simulink model "Final_Tune_of_Bandwidth_PI_Result"  (R2022b)
settings: Solver=FixedStepDiscrete  StartTime=0.0  StopTime=Inf  FixedStep=100e-6  RelTol=1e-3  EnableMultiTasking=on
undefined symbols (not defined in the file): C28x, CPU1, CPU2, CurrentBypassValue, DiscIntNeverNeededParam, Down, GPTRIP1SEL, TZ1, Up
libraries: c2802xlib x20, simulink x16, dspstat3 x10, dspsigops x6, c2837xDlib x5, PID_Lib x5, c280xlib x3, c2000lib x1
(part 2 of 3)

== system Final_Tune_of_Bandwidth_PI_Result/Subsystem1/SVM ==
  Vabc : Inport
  Vdc : Inport  Port=2
  Add : Sum
  Add1 : Sum
  Constant1 : Constant
  Divide : Product  Inputs=*/
  Gain : Gain  Gain=uint32(5000)
  Gain2 : Gain  Gain=0.5
  Gain8 : Gain  Gain=0.5
  Gain9 : Gain  Gain=0.5
  Max : MinMax  Function=max
  Max1 : MinMax
  Saturation : Saturate  UpperLimit=single(2/sqrt(3))  LowerLimit=single(-2/sqrt(3))
  Saturation1 : Saturate  UpperLimit=5000  LowerLimit=0
  Subtract : Sum  Inputs=+-
  Dabc : Outport
  wires:
  Max/1 -> Add/1
  Gain8/1 -> Divide/2
  Add1/1 -> Gain9/1
  Add/1 -> Gain2/1
  Vabc/1 -> Subtract/1, Max1/1, Max/1
  Max1/1 -> Add/2
  Divide/1 -> Saturation/1
  Constant1/1 -> Add1/2
  Gain2/1 -> Subtract/2
  Subtract/1 -> Divide/1
  Gain9/1 -> Gain/1
  Vdc/1 -> Gain8/1
  Saturation/1 -> Add1/1
  Gain/1 -> Saturation1/1
  Saturation1/1 -> Dabc/1

== system Final_Tune_of_Bandwidth_PI_Result/Subsystem1/Start ==
  Data : Inport
  Data_width : Inport  Port=2
  Action Port : ActionPort  ActionPortLabel=if(u1 == 0)
  Bias : Bias  Bias=1  SaturateOnIntegerOverflow=off
  End : Constant  Value=hex2dec('5353')  OutDataTypeStr=uint16
  Mux : Mux  Inputs=2
  Data_out : Outport  VectorParamsAs1DForOutWhenUnconnected=off
  Iteration : Outport  Port=2  VectorParamsAs1DForOutWhenUnconnected=off
  wires:
  End/1 -> Mux/1
  Mux/1 -> Data_out/1
  Data_width/1 -> Bias/1
  Bias/1 -> Iteration/1
  Data/1 -> Mux/2

== system Final_Tune_of_Bandwidth_PI_Result/Subsystem1/Subsystem ==
  PWM1 : Inport
  PWM2 : Inport  Port=2
  PWM3 : Inport  Port=3
  Trip : Inport  Port=4
  Constant12 : Constant  Value=uint32(4999)
  Constant13 : Constant  Value=uint32(0)
  Constant16 : Constant  Value=uint32(4999)
  Constant17 : Constant  Value=uint32(0)
  Constant6 : Constant  Value=uint32(4999)
  Constant7 : Constant  Value=uint32(0)
  Data Type Conversion18 : DataTypeConversion  OutDataTypeStr=uint32  SaturateOnIntegerOverflow=off  RndMeth=Floor
  Data Type Conversion19 : DataTypeConversion  OutDataTypeStr=uint32  SaturateOnIntegerOverflow=off  RndMeth=Floor
  Data Type Conversion5 : DataTypeConversion  OutDataTypeStr=uint32  SaturateOnIntegerOverflow=off  RndMeth=Floor
  From : From
  From1 : From
  From2 : From
  Gain : Gain
  Goto : Goto
  Saturation Dynamic1 : simulink/Discontinuities/Saturation Dynamic  OutMin=[]  OutMax=[]  OutDataTypeStr=Inherit: Same as second input  OutDataType=fixdt(1, 16)  OutScaling=2^-10  DoSatur=off
  Saturation Dynamic2 : simulink/Discontinuities/Saturation Dynamic  OutMin=[]  OutMax=[]  OutDataTypeStr=Inherit: Same as second input  OutDataType=fixdt(1, 16)  OutScaling=2^-10  DoSatur=off
  Saturation Dynamic3 : simulink/Discontinuities/Saturation Dynamic  OutMin=[]  OutMax=[]  OutDataTypeStr=Inherit: Same as second input  OutDataType=fixdt(1, 16)  OutScaling=2^-10  DoSatur=off
  ePWM5 : c2802xlib/ePWM  PwmType=C2000_Type4  useModule=ePWM1  ePWMxLINKTBPRD=Not Linked  periodUnits=Clock cycles  timerSource=Specify via dialog  timerPeriod_clk=5000  timerPeriod_sec=0.0001  tbshadow=Counter equals to zero  countingMode=Up-Down  phaseActiveEnable=Disable  phaseDirection=Count down after sync  phaseActive=0  synchronizationEnable=off  dcaevt1Sync=off  dcbevt1Sync=off  synchronizationOption=Disable  dcbevt1SyncOut=off  dcaevt1SyncOut=off  cmpdSyncOut=off  cmpcSyncOut=off  cmpbSyncOut=off  zeroSyncOut=off  swfSyncOut=off  perSynchronizationOption=Counter equals to period (CTR=PRD)  clockPrescale=1  HSclockPrescale=1  enswap=off  ePWMxAStatus=on  ePWMxAactionLogic1=Do nothing  ePWMxAactionLogic2=Do nothing  ePWMxAactionLogic3=Clear  ePWMxAactionLogic4=Set  ePWMxAactionLogic5=Do nothing  ePWMxAactionLogic6=Do nothing  ePWMxACSFenable=off  ePWMxACSFvalue=Forcing disable  ePWMxASFreload=Zero  ePWMxBStatus=off  ePWMxBactionLogic1=Set  ePWMxBactionLogic2=Clear  ePWMxBactionLogic3=Do nothing  ePWMxBactionLogic4=Do nothing  ePWMxBactionLogic5=Clear  ePWMxBactionLogic6=Set  ePWMxBCSFenable=off  ePWMxBCSFvalue=Forcing disable  ePWMxBSFreload=Zero  ePWNxBOutWay=off  ePWMxLINKCMPA=Not Linked  CMPAUnits=Clock cycles  CMPASource=Input port  CMPAValue_per=50  CMPAValue_clk=0  enCMPAshadow=Counter equals to zero (CTR=Zero)  ePWMxLINKCMPB=Not Linked  CMPBUnits=Clock cycles  CMPBSource=Specify via dialog  CMPBValue_per=50  CMPBValue_clk=0  enCMPBshadow=Counter equals to zero (CTR=Zero)  ePWMxLINKCMPC=Not Linked  CMPCUnits=Clock cycles  CMPCSource=Specify via dialog  CMPCValue_per=50  CMPCValue_clk=0  enCMPCshadow=Counter equals to zero (CTR=Zero)  ePWMxLINKCMPD=Not Linked  CMPDUnits=Clock cycles  CMPDSource=Specify via dialog  CMPDValue_per=50  CMPDValue_clk=32000  enCMPDshadow=Counter equals to zero (CTR=Zero)  enableDBePWMxA=on  enableDBePWMxB=on  enhalfcycle=off  DBpolarity=Active high complementary (AHC)  DBedgeDelay=Positive  DBSource_ePWMxA=ePWMxA  DBSource_ePWMxB=ePWMxA  DBPeriodUnits=Clock cycles  DBperiodSource=Specify via dialog  REDperiod=250  FEDperiod=250  REDperiod_sec=0  FEDperiod_sec=0  LoadModeDBRED=Immediate without using shadow  LoadModeDBFED=Immediate without using shadow  adcstartModuleA=on  adcrequestEventA=First event  adcstartEventA=Digital Compare Module A Event 1 start of conversion (DCAEVT1.soc)  adcstartEventA_type2=Counter equals to period (CTR=PRD)  adcstartModuleB=off  adcrequestEventB=First event  adcstartEventB=Counter equals to zero (CTR=Zero)  adcstartEventB_type2=Counter equals to zero (CTR=Zero)  intEn=off  intPrd=First event  intSel=Counter equals to zero (CTR=Zero)  intSel_type2=Counter equals to zero (CTR=Zero)  hrpe=off  enHRPWM=off  HRPWM_LoadMode=Counter equals to period (CTR=PRD)  HRPWM_CTLMode=Duty or Period control mode  HRPWM_EDGMode=Both edge  hrpeb=off  enHRPWMB=off  HRPWM_LoadModeB=Counter equals to zero (CTR=ZERO)  HRPWM_CTLModeB=Duty or Period control mode  HRPWM_EDGModeB=Both edge  enHRDBRED=off  enHRDBFED=off  enSFO=on  enautoconv=on  chopperEnable=off  chopperFrequency=1  chopperFirstwidth=1  chopperDuty=12.5%  tripZonesource=Input port  tzselOSHT1=off  tzselOSHT2=off  tzselOSHT3=off  tzselOSHDCAEV1=off  tzselOSHDCBEV1=off  tzselCBC1=off  tzselCBC2=off  tzselCBC3=off  tzselCBCDCAEV2=off  tzselCBCDCBEV2=off  tzselOSHT4=off  tzselOSHT5=off  tzselOSHT6=off  tzselCBC4=off  tzselCBC5=off  tzselCBC6=off  enTzOstIntr=off  enTzCbcIntr=off  enTzDCAEVT1Intr=off  enTzDCAEVT2Intr=off  enTzDCBEVT1Intr=off  enTzDCBEVT2Intr=off  ePWMxAforced=Low  ePWMxBforced=Low  DCAEVT1forced=No action  DCBEVT1forced=No action  DCAEVT2forced=No action  DCBEVT2forced=No action  dcah=Trip Zone 1 input (TZ1)  dcal=Trip Zone 2 input (TZ2)  dcbh=Trip Zone 1 input (TZ1)  dcbl=Trip Zone 2 input (TZ2)  dcah_type2=GPTRIP1SEL/(TZ1)  dcal_type2=GPTRIP1SEL/(TZ1)  dcbh_type2=GPTRIP1SEL/(TZ1)  dcbl_type2=GPTRIP1SEL/(TZ1)  gendcaevt1=Event disabled  gendcaevt2=Event disabled  gendcbevt1=Event disabled  gendcbevt2=Event disabled  dcaevt1src=DCAEVT1 with sync  dcaevt2src=DCAEVT2 with sync  dcbevt1src=DCBEVT1 with sync  dcbevt2src=DCBEVT2 with sync  pulsesel=Counter equals to zero (CTR=Zero)  blankinv=off  blankoffset=0  blankwidth=0  evsrcsel=Filtered version of DCAEVT1 (DCAEVT1FILT)  encape=off
  ePWM6 : c2802xlib/ePWM  PwmType=C2000_Type4  useModule=ePWM2  ePWMxLINKTBPRD=Not Linked  periodUnits=Clock cycles  timerSource=Specify via dialog  timerPeriod_clk=5000  timerPeriod_sec=0.0001  tbshadow=Counter equals to zero  countingMode=Up-Down  phaseActiveEnable=Disable  phaseDirection=Count down after sync  phaseActive=0  synchronizationEnable=off  dcaevt1Sync=off  dcbevt1Sync=off  synchronizationOption=Disable  dcbevt1SyncOut=off  dcaevt1SyncOut=off  cmpdSyncOut=off  cmpcSyncOut=off  cmpbSyncOut=off  zeroSyncOut=off  swfSyncOut=off  perSynchronizationOption=Counter equals to period (CTR=PRD)  clockPrescale=1  HSclockPrescale=1  enswap=off  ePWMxAStatus=on  ePWMxAactionLogic1=Do nothing  ePWMxAactionLogic2=Do nothing  ePWMxAactionLogic3=Clear  ePWMxAactionLogic4=Set  ePWMxAactionLogic5=Do nothing  ePWMxAactionLogic6=Do nothing  ePWMxACSFenable=off  ePWMxACSFvalue=Forcing disable  ePWMxASFreload=Zero  ePWMxBStatus=off  ePWMxBactionLogic1=Set  ePWMxBactionLogic2=Clear  ePWMxBactionLogic3=Do nothing  ePWMxBactionLogic4=Do nothing  ePWMxBactionLogic5=Clear  ePWMxBactionLogic6=Set  ePWMxBCSFenable=off  ePWMxBCSFvalue=Forcing disable  ePWMxBSFreload=Zero  ePWNxBOutWay=off  ePWMxLINKCMPA=Not Linked  CMPAUnits=Clock cycles  CMPASource=Input port  CMPAValue_per=50  CMPAValue_clk=0  enCMPAshadow=Counter equals to zero (CTR=Zero)  ePWMxLINKCMPB=Not Linked  CMPBUnits=Clock cycles  CMPBSource=Specify via dialog  CMPBValue_per=50  CMPBValue_clk=0  enCMPBshadow=Counter equals to zero (CTR=Zero)  ePWMxLINKCMPC=Not Linked  CMPCUnits=Clock cycles  CMPCSource=Specify via dialog  CMPCValue_per=50  CMPCValue_clk=0  enCMPCshadow=Counter equals to zero (CTR=Zero)  ePWMxLINKCMPD=Not Linked  CMPDUnits=Clock cycles  CMPDSource=Specify via dialog  CMPDValue_per=50  CMPDValue_clk=32000  enCMPDshadow=Counter equals to zero (CTR=Zero)  enableDBePWMxA=on  enableDBePWMxB=on  enhalfcycle=off  DBpolarity=Active high complementary (AHC)  DBedgeDelay=Positive  DBSource_ePWMxA=ePWMxA  DBSource_ePWMxB=ePWMxA  DBPeriodUnits=Clock cycles  DBperiodSource=Specify via dialog  REDperiod=250  FEDperiod=250  REDperiod_sec=0  FEDperiod_sec=0  LoadModeDBRED=Immediate without using shadow  LoadModeDBFED=Immediate without using shadow  adcstartModuleA=off  adcrequestEventA=First event  adcstartEventA=Digital Compare Module A Event 1 start of conversion (DCAEVT1.soc)  adcstartEventA_type2=Counter equals to zero (CTR=Zero)  adcstartModuleB=off  adcrequestEventB=First event  adcstartEventB=Counter equals to zero (CTR=Zero)  adcstartEventB_type2=Counter equals to zero (CTR=Zero)  intEn=off  intPrd=First event  intSel=Counter equals to zero (CTR=Zero)  intSel_type2=Counter equals to zero (CTR=Zero)  hrpe=off  enHRPWM=off  HRPWM_LoadMode=Counter equals to period (CTR=PRD)  HRPWM_CTLMode=Duty or Period control mode  HRPWM_EDGMode=Both edge  hrpeb=off  enHRPWMB=off  HRPWM_LoadModeB=Counter equals to zero (CTR=ZERO)  HRPWM_CTLModeB=Duty or Period control mode  HRPWM_EDGModeB=Both edge  enHRDBRED=off  enHRDBFED=off  enSFO=on  enautoconv=on  chopperEnable=off  chopperFrequency=1  chopperFirstwidth=1  chopperDuty=12.5%  tripZonesource=Input port  tzselOSHT1=off  tzselOSHT2=off  tzselOSHT3=off  tzselOSHDCAEV1=off  tzselOSHDCBEV1=off  tzselCBC1=off  tzselCBC2=off  tzselCBC3=off  tzselCBCDCAEV2=off  tzselCBCDCBEV2=off  tzselOSHT4=off  tzselOSHT5=off  tzselOSHT6=off  tzselCBC4=off  tzselCBC5=off  tzselCBC6=off  enTzOstIntr=off  enTzCbcIntr=off  enTzDCAEVT1Intr=off  enTzDCAEVT2Intr=off  enTzDCBEVT1Intr=off  enTzDCBEVT2Intr=off  ePWMxAforced=Low  ePWMxBforced=Low  DCAEVT1forced=No action  DCBEVT1forced=No action  DCAEVT2forced=No action  DCBEVT2forced=No action  dcah=Trip Zone 1 input (TZ1)  dcal=Trip Zone 2 input (TZ2)  dcbh=Trip Zone 1 input (TZ1)  dcbl=Trip Zone 2 input (TZ2)  dcah_type2=GPTRIP1SEL/(TZ1)  dcal_type2=GPTRIP1SEL/(TZ1)  dcbh_type2=GPTRIP1SEL/(TZ1)  dcbl_type2=GPTRIP1SEL/(TZ1)  gendcaevt1=Event disabled  gendcaevt2=Event disabled  gendcbevt1=Event disabled  gendcbevt2=Event disabled  dcaevt1src=DCAEVT1 with sync  dcaevt2src=DCAEVT2 with sync  dcbevt1src=DCBEVT1 with sync  dcbevt2src=DCBEVT2 with sync  pulsesel=Counter equals to zero (CTR=Zero)  blankinv=off  blankoffset=0  blankwidth=0  evsrcsel=Filtered version of DCAEVT1 (DCAEVT1FILT)  encape=off
  ePWM7 : c2802xlib/ePWM  PwmType=C2000_Type4  useModule=ePWM3  ePWMxLINKTBPRD=Not Linked  periodUnits=Clock cycles  timerSource=Specify via dialog  timerPeriod_clk=5000  timerPeriod_sec=0.0001  tbshadow=Counter equals to zero  countingMode=Up-Down  phaseActiveEnable=Disable  phaseDirection=Count down after sync  phaseActive=0  synchronizationEnable=off  dcaevt1Sync=off  dcbevt1Sync=off  synchronizationOption=Disable  dcbevt1SyncOut=off  dcaevt1SyncOut=off  cmpdSyncOut=off  cmpcSyncOut=off  cmpbSyncOut=off  zeroSyncOut=off  swfSyncOut=off  perSynchronizationOption=Counter equals to period (CTR=PRD)  clockPrescale=1  HSclockPrescale=1  enswap=off  ePWMxAStatus=on  ePWMxAactionLogic1=Do nothing  ePWMxAactionLogic2=Do nothing  ePWMxAactionLogic3=Clear  ePWMxAactionLogic4=Set  ePWMxAactionLogic5=Do nothing  ePWMxAactionLogic6=Do nothing  ePWMxACSFenable=off  ePWMxACSFvalue=Forcing disable  ePWMxASFreload=Zero  ePWMxBStatus=off  ePWMxBactionLogic1=Set  ePWMxBactionLogic2=Clear  ePWMxBactionLogic3=Do nothing  ePWMxBactionLogic4=Do nothing  ePWMxBactionLogic5=Clear  ePWMxBactionLogic6=Set  ePWMxBCSFenable=off  ePWMxBCSFvalue=Forcing disable  ePWMxBSFreload=Zero  ePWNxBOutWay=off  ePWMxLINKCMPA=Not Linked  CMPAUnits=Clock cycles  CMPASource=Input port  CMPAValue_per=50  CMPAValue_clk=0  enCMPAshadow=Counter equals to zero (CTR=Zero)  ePWMxLINKCMPB=Not Linked  CMPBUnits=Clock cycles  CMPBSource=Specify via dialog  CMPBValue_per=50  CMPBValue_clk=0  enCMPBshadow=Counter equals to zero (CTR=Zero)  ePWMxLINKCMPC=Not Linked  CMPCUnits=Clock cycles  CMPCSource=Specify via dialog  CMPCValue_per=50  CMPCValue_clk=0  enCMPCshadow=Counter equals to zero (CTR=Zero)  ePWMxLINKCMPD=Not Linked  CMPDUnits=Clock cycles  CMPDSource=Specify via dialog  CMPDValue_per=50  CMPDValue_clk=32000  enCMPDshadow=Counter equals to zero (CTR=Zero)  enableDBePWMxA=on  enableDBePWMxB=on  enhalfcycle=off  DBpolarity=Active high complementary (AHC)  DBedgeDelay=Positive  DBSource_ePWMxA=ePWMxA  DBSource_ePWMxB=ePWMxA  DBPeriodUnits=Clock cycles  DBperiodSource=Specify via dialog  REDperiod=250  FEDperiod=250  REDperiod_sec=0  FEDperiod_sec=0  LoadModeDBRED=Immediate without using shadow  LoadModeDBFED=Immediate without using shadow  adcstartModuleA=off  adcrequestEventA=First event  adcstartEventA=Digital Compare Module A Event 1 start of conversion (DCAEVT1.soc)  adcstartEventA_type2=Counter equals to zero (CTR=Zero)  adcstartModuleB=off  adcrequestEventB=First event  adcstartEventB=Counter equals to zero (CTR=Zero)  adcstartEventB_type2=Counter equals to zero (CTR=Zero)  intEn=off  intPrd=First event  intSel=Counter equals to zero (CTR=Zero)  intSel_type2=Counter equals to zero (CTR=Zero)  hrpe=off  enHRPWM=off  HRPWM_LoadMode=Counter equals to period (CTR=PRD)  HRPWM_CTLMode=Duty or Period control mode  HRPWM_EDGMode=Both edge  hrpeb=off  enHRPWMB=off  HRPWM_LoadModeB=Counter equals to zero (CTR=ZERO)  HRPWM_CTLModeB=Duty or Period control mode  HRPWM_EDGModeB=Both edge  enHRDBRED=off  enHRDBFED=off  enSFO=on  enautoconv=on  chopperEnable=off  chopperFrequency=1  chopperFirstwidth=1  chopperDuty=12.5%  tripZonesource=Input port  tzselOSHT1=off  tzselOSHT2=off  tzselOSHT3=off  tzselOSHDCAEV1=off  tzselOSHDCBEV1=off  tzselCBC1=off  tzselCBC2=off  tzselCBC3=off  tzselCBCDCAEV2=off  tzselCBCDCBEV2=off  tzselOSHT4=off  tzselOSHT5=off  tzselOSHT6=off  tzselCBC4=off  tzselCBC5=off  tzselCBC6=off  enTzOstIntr=off  enTzCbcIntr=off  enTzDCAEVT1Intr=off  enTzDCAEVT2Intr=off  enTzDCBEVT1Intr=off  enTzDCBEVT2Intr=off  ePWMxAforced=Low  ePWMxBforced=Low  DCAEVT1forced=No action  DCBEVT1forced=No action  DCAEVT2forced=No action  DCBEVT2forced=No action  dcah=Trip Zone 1 input (TZ1)  dcal=Trip Zone 2 input (TZ2)  dcbh=Trip Zone 1 input (TZ1)  dcbl=Trip Zone 2 input (TZ2)  dcah_type2=GPTRIP1SEL/(TZ1)  dcal_type2=GPTRIP1SEL/(TZ1)  dcbh_type2=GPTRIP1SEL/(TZ1)  dcbl_type2=GPTRIP1SEL/(TZ1)  gendcaevt1=Event disabled  gendcaevt2=Event disabled  gendcbevt1=Event disabled  gendcbevt2=Event disabled  dcaevt1src=DCAEVT1 with sync  dcaevt2src=DCAEVT2 with sync  dcbevt1src=DCBEVT1 with sync  dcbevt2src=DCBEVT2 with sync  pulsesel=Counter equals to zero (CTR=Zero)  blankinv=off  blankoffset=0  blankwidth=0  evsrcsel=Filtered version of DCAEVT1 (DCAEVT1FILT)  encape=off
  wires:
  Data Type Conversion5/1 -> ePWM5/1
  Constant13/1 -> Saturation Dynamic3/3
  Constant6/1 -> Saturation Dynamic1/1
  Constant12/1 -> Saturation Dynamic3/1
  Constant7/1 -> Saturation Dynamic1/3
  Saturation Dynamic1/1 -> Data Type Conversion5/1
  Constant16/1 -> Saturation Dynamic2/1
  Data Type Conversion18/1 -> ePWM6/1
  Data Type Conversion19/1 -> ePWM7/1
  Saturation Dynamic3/1 -> Data Type Conversion19/1
  Constant17/1 -> Saturation Dynamic2/3
  Saturation Dynamic2/1 -> Data Type Conversion18/1
  PWM1/1 -> Saturation Dynamic1/2
  PWM3/1 -> Saturation Dynamic3/2
  PWM2/1 -> Saturation Dynamic2/2
  From/1 -> ePWM5/2
  From1/1 -> ePWM6/2
  From2/1 -> ePWM7/2
  Trip/1 -> Gain/1
  Gain/1 -> Goto/1

== system Final_Tune_of_Bandwidth_PI_Result/Subsystem1/Subsystem1 ==
  In1 : Inport
  In2 : Inport  Port=2
  Enable : EnablePort  StatesWhenEnabling=reset
  Add : Sum
  Add3 : Sum
  Bus Creator : BusCreator  Inputs=2
  Bus Selector1 : BusSelector  OutputSignals=signal1,signal2
  CodeGeneration : Subsystem  TreatAsAtomicUnit=on
  Constant3 : Constant  Value=10  OutDataTypeStr=single
  Counter Limited : simulink/Sources/Counter Limited  uplimit=599  tsamp=-1
  Data : Subsystem  TreatAsAtomicUnit=on
  Data_Conditioning : Subsystem
  End : Subsystem  TreatAsAtomicUnit=on
  Gain6 : Gain  Gain=1000  OutDataTypeStr=single
  Gain7 : Gain  Gain=1000  OutDataTypeStr=single
  If : If  IfExpression=u1 == 0  ElseIfExpressions=u1 == 599
  Merge : Merge  Inputs=3
  Merge1 : Merge  Inputs=3
  Mux : Mux  Inputs=2
  Mux1 : Mux  Inputs=2
  Start : Subsystem  TreatAsAtomicUnit=on
  Width : Width  OutDataTypeMode=All ports same datatype  DataType=uint16
  wires:
  Start/2(Iteration) -> Merge1/1
  Constant3/1 -> Add/2, Add3/1
  Counter Limited/1 -> If/1
  Data_Conditioning/1(Out1) -> Width/1, Start/1(Data), End/1(Data), Data/1(Data)
  End/1(Data_out) -> Merge/2
  End/2(Iteration) -> Merge1/2
  If/3 -> Data/Action
  Add/1 -> Gain6/1
  Data/2(Iteration) -> Merge1/3
  Merge1/1 -> Mux/2  "SCI_Tx_Iteration"
  Bus Selector1/1 -> Add/1  "<signal1>"
  Start/1(Data_out) -> Merge/1
  Add3/1 -> Gain7/1
  Mux1/1 -> Data_Conditioning/1(In1)
  In1/1 -> Bus Creator/1
  Merge/1 -> Mux/1  "SCI_Tx_Data"
  If/2 -> End/Action
  Data/1(Data_out) -> Merge/3
  Bus Creator/1 -> Bus Selector1/1
  Width/1 -> Start/2(Data_width), Data/2(Data_width), End/2(Data_width)
  Mux/1 -> CodeGeneration/1(Input)
  In2/1 -> Bus Creator/2
  Gain7/1 -> Mux1/2
  Bus Selector1/2 -> Add3/2  "<signal2>"
  If/1 -> Start/Action
  Gain6/1 -> Mux1/1

== system Final_Tune_of_Bandwidth_PI_Result/Subsystem1/Subsystem2 ==
  PWM1 : Inport
  PWM2 : Inport  Port=2
  PWM3 : Inport  Port=3
  Trip : Inport  Port=4
  Constant12 : Constant  Value=uint32(4999)
  Constant13 : Constant  Value=uint32(0)
  Constant16 : Constant  Value=uint32(4999)
  Constant17 : Constant  Value=uint32(0)
  Constant6 : Constant  Value=uint32(4999)
  Constant7 : Constant  Value=uint32(0)
  Data Type Conversion18 : DataTypeConversion  OutDataTypeStr=uint32  SaturateOnIntegerOverflow=off  RndMeth=Floor
  Data Type Conversion19 : DataTypeConversion  OutDataTypeStr=uint32  SaturateOnIntegerOverflow=off  RndMeth=Floor
  Data Type Conversion5 : DataTypeConversion  OutDataTypeStr=uint32  SaturateOnIntegerOverflow=off  RndMeth=Floor
  From : From
  From1 : From
  From2 : From
  Gain : Gain
  Goto : Goto
  Saturation Dynamic1 : simulink/Discontinuities/Saturation Dynamic  OutMin=[]  OutMax=[]  OutDataTypeStr=Inherit: Same as second input  OutDataType=fixdt(1, 16)  OutScaling=2^-10  DoSatur=off
  Saturation Dynamic2 : simulink/Discontinuities/Saturation Dynamic  OutMin=[]  OutMax=[]  OutDataTypeStr=Inherit: Same as second input  OutDataType=fixdt(1, 16)  OutScaling=2^-10  DoSatur=off
  Saturation Dynamic3 : simulink/Discontinuities/Saturation Dynamic  OutMin=[]  OutMax=[]  OutDataTypeStr=Inherit: Same as second input  OutDataType=fixdt(1, 16)  OutScaling=2^-10  DoSatur=off
  ePWM5 : c2802xlib/ePWM  PwmType=C2000_Type4  useModule=ePWM1  ePWMxLINKTBPRD=Not Linked  periodUnits=Clock cycles  timerSource=Specify via dialog  timerPeriod_clk=5000  timerPeriod_sec=0.0001  tbshadow=Counter equals to zero  countingMode=Up-Down  phaseActiveEnable=Disable  phaseDirection=Count down after sync  phaseActive=0  synchronizationEnable=off  dcaevt1Sync=off  dcbevt1Sync=off  synchronizationOption=Disable  dcbevt1SyncOut=off  dcaevt1SyncOut=off  cmpdSyncOut=off  cmpcSyncOut=off  cmpbSyncOut=off  zeroSyncOut=off  swfSyncOut=off  perSynchronizationOption=Counter equals to period (CTR=PRD)  clockPrescale=1  HSclockPrescale=1  enswap=off  ePWMxAStatus=on  ePWMxAactionLogic1=Do nothing  ePWMxAactionLogic2=Do nothing  ePWMxAactionLogic3=Clear  ePWMxAactionLogic4=Set  ePWMxAactionLogic5=Do nothing  ePWMxAactionLogic6=Do nothing  ePWMxACSFenable=off  ePWMxACSFvalue=Forcing disable  ePWMxASFreload=Zero  ePWMxBStatus=off  ePWMxBactionLogic1=Set  ePWMxBactionLogic2=Clear  ePWMxBactionLogic3=Do nothing  ePWMxBactionLogic4=Do nothing  ePWMxBactionLogic5=Clear  ePWMxBactionLogic6=Set  ePWMxBCSFenable=off  ePWMxBCSFvalue=Forcing disable  ePWMxBSFreload=Zero  ePWNxBOutWay=off  ePWMxLINKCMPA=Not Linked  CMPAUnits=Clock cycles  CMPASource=Input port  CMPAValue_per=50  CMPAValue_clk=0  enCMPAshadow=Counter equals to zero (CTR=Zero)  ePWMxLINKCMPB=Not Linked  CMPBUnits=Clock cycles  CMPBSource=Specify via dialog  CMPBValue_per=50  CMPBValue_clk=0  enCMPBshadow=Counter equals to zero (CTR=Zero)  ePWMxLINKCMPC=Not Linked  CMPCUnits=Clock cycles  CMPCSource=Specify via dialog  CMPCValue_per=50  CMPCValue_clk=0  enCMPCshadow=Counter equals to zero (CTR=Zero)  ePWMxLINKCMPD=Not Linked  CMPDUnits=Clock cycles  CMPDSource=Specify via dialog  CMPDValue_per=50  CMPDValue_clk=32000  enCMPDshadow=Counter equals to zero (CTR=Zero)  enableDBePWMxA=on  enableDBePWMxB=on  enhalfcycle=off  DBpolarity=Active high complementary (AHC)  DBedgeDelay=Positive  DBSource_ePWMxA=ePWMxA  DBSource_ePWMxB=ePWMxA  DBPeriodUnits=Seconds  DBperiodSource=Specify via dialog  REDperiod=250  FEDperiod=250  REDperiod_sec=500e-9  FEDperiod_sec=500e-9  LoadModeDBRED=Immediate without using shadow  LoadModeDBFED=Immediate without using shadow  adcstartModuleA=on  adcrequestEventA=First event  adcstartEventA=Digital Compare Module A Event 1 start of conversion (DCAEVT1.soc)  adcstartEventA_type2=Counter equals to period (CTR=PRD)  adcstartModuleB=off  adcrequestEventB=First event  adcstartEventB=Counter equals to zero (CTR=Zero)  adcstartEventB_type2=Counter equals to zero (CTR=Zero)  intEn=off  intPrd=First event  intSel=Counter equals to zero (CTR=Zero)  intSel_type2=Counter equals to zero (CTR=Zero)  hrpe=off  enHRPWM=off  HRPWM_LoadMode=Counter equals to period (CTR=PRD)  HRPWM_CTLMode=Duty or Period control mode  HRPWM_EDGMode=Both edge  hrpeb=off  enHRPWMB=off  HRPWM_LoadModeB=Counter equals to zero (CTR=ZERO)  HRPWM_CTLModeB=Duty or Period control mode  HRPWM_EDGModeB=Both edge  enHRDBRED=off  enHRDBFED=off  enSFO=on  enautoconv=on  chopperEnable=off  chopperFrequency=1  chopperFirstwidth=1  chopperDuty=12.5%  tripZonesource=Input port  tzselOSHT1=off  tzselOSHT2=off  tzselOSHT3=off  tzselOSHDCAEV1=off  tzselOSHDCBEV1=off  tzselCBC1=off  tzselCBC2=off  tzselCBC3=off  tzselCBCDCAEV2=off  tzselCBCDCBEV2=off  tzselOSHT4=off  tzselOSHT5=off  tzselOSHT6=off  tzselCBC4=off  tzselCBC5=off  tzselCBC6=off  enTzOstIntr=off  enTzCbcIntr=off  enTzDCAEVT1Intr=off  enTzDCAEVT2Intr=off  enTzDCBEVT1Intr=off  enTzDCBEVT2Intr=off  ePWMxAforced=Low  ePWMxBforced=Low  DCAEVT1forced=No action  DCBEVT1forced=No action  DCAEVT2forced=No action  DCBEVT2forced=No action  dcah=Trip Zone 1 input (TZ1)  dcal=Trip Zone 2 input (TZ2)  dcbh=Trip Zone 1 input (TZ1)  dcbl=Trip Zone 2 input (TZ2)  dcah_type2=GPTRIP1SEL/(TZ1)  dcal_type2=GPTRIP1SEL/(TZ1)  dcbh_type2=GPTRIP1SEL/(TZ1)  dcbl_type2=GPTRIP1SEL/(TZ1)  gendcaevt1=Event disabled  gendcaevt2=Event disabled  gendcbevt1=Event disabled  gendcbevt2=Event disabled  dcaevt1src=DCAEVT1 with sync  dcaevt2src=DCAEVT2 with sync  dcbevt1src=DCBEVT1 with sync  dcbevt2src=DCBEVT2 with sync  pulsesel=Counter equals to zero (CTR=Zero)  blankinv=off  blankoffset=0  blankwidth=0  evsrcsel=Filtered version of DCAEVT1 (DCAEVT1FILT)  encape=off
  ePWM6 : c2802xlib/ePWM  PwmType=C2000_Type4  useModule=ePWM2  ePWMxLINKTBPRD=Not Linked  periodUnits=Clock cycles  timerSource=Specify via dialog  timerPeriod_clk=5000  timerPeriod_sec=0.0001  tbshadow=Counter equals to zero  countingMode=Up-Down  phaseActiveEnable=Disable  phaseDirection=Count down after sync  phaseActive=0  synchronizationEnable=off  dcaevt1Sync=off  dcbevt1Sync=off  synchronizationOption=Disable  dcbevt1SyncOut=off  dcaevt1SyncOut=off  cmpdSyncOut=off  cmpcSyncOut=off  cmpbSyncOut=off  zeroSyncOut=off  swfSyncOut=off  perSynchronizationOption=Counter equals to period (CTR=PRD)  clockPrescale=1  HSclockPrescale=1  enswap=off  ePWMxAStatus=on  ePWMxAactionLogic1=Do nothing  ePWMxAactionLogic2=Do nothing  ePWMxAactionLogic3=Clear  ePWMxAactionLogic4=Set  ePWMxAactionLogic5=Do nothing  ePWMxAactionLogic6=Do nothing  ePWMxACSFenable=off  ePWMxACSFvalue=Forcing disable  ePWMxASFreload=Zero  ePWMxBStatus=off  ePWMxBactionLogic1=Set  ePWMxBactionLogic2=Clear  ePWMxBactionLogic3=Do nothing  ePWMxBactionLogic4=Do nothing  ePWMxBactionLogic5=Clear  ePWMxBactionLogic6=Set  ePWMxBCSFenable=off  ePWMxBCSFvalue=Forcing disable  ePWMxBSFreload=Zero  ePWNxBOutWay=off  ePWMxLINKCMPA=Not Linked  CMPAUnits=Clock cycles  CMPASource=Input port  CMPAValue_per=50  CMPAValue_clk=0  enCMPAshadow=Counter equals to zero (CTR=Zero)  ePWMxLINKCMPB=Not Linked  CMPBUnits=Clock cycles  CMPBSource=Specify via dialog  CMPBValue_per=50  CMPBValue_clk=0  enCMPBshadow=Counter equals to zero (CTR=Zero)  ePWMxLINKCMPC=Not Linked  CMPCUnits=Clock cycles  CMPCSource=Specify via dialog  CMPCValue_per=50  CMPCValue_clk=0  enCMPCshadow=Counter equals to zero (CTR=Zero)  ePWMxLINKCMPD=Not Linked  CMPDUnits=Clock cycles  CMPDSource=Specify via dialog  CMPDValue_per=50  CMPDValue_clk=32000  enCMPDshadow=Counter equals to zero (CTR=Zero)  enableDBePWMxA=on  enableDBePWMxB=on  enhalfcycle=off  DBpolarity=Active high complementary (AHC)  DBedgeDelay=Positive  DBSource_ePWMxA=ePWMxA  DBSource_ePWMxB=ePWMxA  DBPeriodUnits=Seconds  DBperiodSource=Specify via dialog  REDperiod=250  FEDperiod=250  REDperiod_sec=500e-9  FEDperiod_sec=500e-9  LoadModeDBRED=Immediate without using shadow  LoadModeDBFED=Immediate without using shadow  adcstartModuleA=off  adcrequestEventA=First event  adcstartEventA=Digital Compare Module A Event 1 start of conversion (DCAEVT1.soc)  adcstartEventA_type2=Counter equals to zero (CTR=Zero)  adcstartModuleB=off  adcrequestEventB=First event  adcstartEventB=Counter equals to zero (CTR=Zero)  adcstartEventB_type2=Counter equals to zero (CTR=Zero)  intEn=off  intPrd=First event  intSel=Counter equals to zero (CTR=Zero)  intSel_type2=Counter equals to zero (CTR=Zero)  hrpe=off  enHRPWM=off  HRPWM_LoadMode=Counter equals to period (CTR=PRD)  HRPWM_CTLMode=Duty or Period control mode  HRPWM_EDGMode=Both edge  hrpeb=off  enHRPWMB=off  HRPWM_LoadModeB=Counter equals to zero (CTR=ZERO)  HRPWM_CTLModeB=Duty or Period control mode  HRPWM_EDGModeB=Both edge  enHRDBRED=off  enHRDBFED=off  enSFO=on  enautoconv=on  chopperEnable=off  chopperFrequency=1  chopperFirstwidth=1  chopperDuty=12.5%  tripZonesource=Input port  tzselOSHT1=off  tzselOSHT2=off  tzselOSHT3=off  tzselOSHDCAEV1=off  tzselOSHDCBEV1=off  tzselCBC1=off  tzselCBC2=off  tzselCBC3=off  tzselCBCDCAEV2=off  tzselCBCDCBEV2=off  tzselOSHT4=off  tzselOSHT5=off  tzselOSHT6=off  tzselCBC4=off  tzselCBC5=off  tzselCBC6=off  enTzOstIntr=off  enTzCbcIntr=off  enTzDCAEVT1Intr=off  enTzDCAEVT2Intr=off  enTzDCBEVT1Intr=off  enTzDCBEVT2Intr=off  ePWMxAforced=Low  ePWMxBforced=Low  DCAEVT1forced=No action  DCBEVT1forced=No action  DCAEVT2forced=No action  DCBEVT2forced=No action  dcah=Trip Zone 1 input (TZ1)  dcal=Trip Zone 2 input (TZ2)  dcbh=Trip Zone 1 input (TZ1)  dcbl=Trip Zone 2 input (TZ2)  dcah_type2=GPTRIP1SEL/(TZ1)  dcal_type2=GPTRIP1SEL/(TZ1)  dcbh_type2=GPTRIP1SEL/(TZ1)  dcbl_type2=GPTRIP1SEL/(TZ1)  gendcaevt1=Event disabled  gendcaevt2=Event disabled  gendcbevt1=Event disabled  gendcbevt2=Event disabled  dcaevt1src=DCAEVT1 with sync  dcaevt2src=DCAEVT2 with sync  dcbevt1src=DCBEVT1 with sync  dcbevt2src=DCBEVT2 with sync  pulsesel=Counter equals to zero (CTR=Zero)  blankinv=off  blankoffset=0  blankwidth=0  evsrcsel=Filtered version of DCAEVT1 (DCAEVT1FILT)  encape=off
  ePWM7 : c2802xlib/ePWM  PwmType=C2000_Type4  useModule=ePWM3  ePWMxLINKTBPRD=Not Linked  periodUnits=Clock cycles  timerSource=Specify via dialog  timerPeriod_clk=5000  timerPeriod_sec=0.0001  tbshadow=Counter equals to zero  countingMode=Up-Down  phaseActiveEnable=Disable  phaseDirection=Count down after sync  phaseActive=0  synchronizationEnable=off  dcaevt1Sync=off  dcbevt1Sync=off  synchronizationOption=Disable  dcbevt1SyncOut=off  dcaevt1SyncOut=off  cmpdSyncOut=off  cmpcSyncOut=off  cmpbSyncOut=off  zeroSyncOut=off  swfSyncOut=off  perSynchronizationOption=Counter equals to period (CTR=PRD)  clockPrescale=1  HSclockPrescale=1  enswap=off  ePWMxAStatus=on  ePWMxAactionLogic1=Do nothing  ePWMxAactionLogic2=Do nothing  ePWMxAactionLogic3=Clear  ePWMxAactionLogic4=Set  ePWMxAactionLogic5=Do nothing  ePWMxAactionLogic6=Do nothing  ePWMxACSFenable=off  ePWMxACSFvalue=Forcing disable  ePWMxASFreload=Zero  ePWMxBStatus=off  ePWMxBactionLogic1=Set  ePWMxBactionLogic2=Clear  ePWMxBactionLogic3=Do nothing  ePWMxBactionLogic4=Do nothing  ePWMxBactionLogic5=Clear  ePWMxBactionLogic6=Set  ePWMxBCSFenable=off  ePWMxBCSFvalue=Forcing disable  ePWMxBSFreload=Zero  ePWNxBOutWay=off  ePWMxLINKCMPA=Not Linked  CMPAUnits=Clock cycles  CMPASource=Input port  CMPAValue_per=50  CMPAValue_clk=0  enCMPAshadow=Counter equals to zero (CTR=Zero)  ePWMxLINKCMPB=Not Linked  CMPBUnits=Clock cycles  CMPBSource=Specify via dialog  CMPBValue_per=50  CMPBValue_clk=0  enCMPBshadow=Counter equals to zero (CTR=Zero)  ePWMxLINKCMPC=Not Linked  CMPCUnits=Clock cycles  CMPCSource=Specify via dialog  CMPCValue_per=50  CMPCValue_clk=0  enCMPCshadow=Counter equals to zero (CTR=Zero)  ePWMxLINKCMPD=Not Linked  CMPDUnits=Clock cycles  CMPDSource=Specify via dialog  CMPDValue_per=50  CMPDValue_clk=32000  enCMPDshadow=Counter equals to zero (CTR=Zero)  enableDBePWMxA=on  enableDBePWMxB=on  enhalfcycle=off  DBpolarity=Active high complementary (AHC)  DBedgeDelay=Positive  DBSource_ePWMxA=ePWMxA  DBSource_ePWMxB=ePWMxA  DBPeriodUnits=Seconds  DBperiodSource=Specify via dialog  REDperiod=250  FEDperiod=250  REDperiod_sec=500e-9  FEDperiod_sec=500e-9  LoadModeDBRED=Immediate without using shadow  LoadModeDBFED=Immediate without using shadow  adcstartModuleA=off  adcrequestEventA=First event  adcstartEventA=Digital Compare Module A Event 1 start of conversion (DCAEVT1.soc)  adcstartEventA_type2=Counter equals to zero (CTR=Zero)  adcstartModuleB=off  adcrequestEventB=First event  adcstartEventB=Counter equals to zero (CTR=Zero)  adcstartEventB_type2=Counter equals to zero (CTR=Zero)  intEn=off  intPrd=First event  intSel=Counter equals to zero (CTR=Zero)  intSel_type2=Counter equals to zero (CTR=Zero)  hrpe=off  enHRPWM=off  HRPWM_LoadMode=Counter equals to period (CTR=PRD)  HRPWM_CTLMode=Duty or Period control mode  HRPWM_EDGMode=Both edge  hrpeb=off  enHRPWMB=off  HRPWM_LoadModeB=Counter equals to zero (CTR=ZERO)  HRPWM_CTLModeB=Duty or Period control mode  HRPWM_EDGModeB=Both edge  enHRDBRED=off  enHRDBFED=off  enSFO=on  enautoconv=on  chopperEnable=off  chopperFrequency=1  chopperFirstwidth=1  chopperDuty=12.5%  tripZonesource=Input port  tzselOSHT1=off  tzselOSHT2=off  tzselOSHT3=off  tzselOSHDCAEV1=off  tzselOSHDCBEV1=off  tzselCBC1=off  tzselCBC2=off  tzselCBC3=off  tzselCBCDCAEV2=off  tzselCBCDCBEV2=off  tzselOSHT4=off  tzselOSHT5=off  tzselOSHT6=off  tzselCBC4=off  tzselCBC5=off  tzselCBC6=off  enTzOstIntr=off  enTzCbcIntr=off  enTzDCAEVT1Intr=off  enTzDCAEVT2Intr=off  enTzDCBEVT1Intr=off  enTzDCBEVT2Intr=off  ePWMxAforced=Low  ePWMxBforced=Low  DCAEVT1forced=No action  DCBEVT1forced=No action  DCAEVT2forced=No action  DCBEVT2forced=No action  dcah=Trip Zone 1 input (TZ1)  dcal=Trip Zone 2 input (TZ2)  dcbh=Trip Zone 1 input (TZ1)  dcbl=Trip Zone 2 input (TZ2)  dcah_type2=GPTRIP1SEL/(TZ1)  dcal_type2=GPTRIP1SEL/(TZ1)  dcbh_type2=GPTRIP1SEL/(TZ1)  dcbl_type2=GPTRIP1SEL/(TZ1)  gendcaevt1=Event disabled  gendcaevt2=Event disabled  gendcbevt1=Event disabled  gendcbevt2=Event disabled  dcaevt1src=DCAEVT1 with sync  dcaevt2src=DCAEVT2 with sync  dcbevt1src=DCBEVT1 with sync  dcbevt2src=DCBEVT2 with sync  pulsesel=Counter equals to zero (CTR=Zero)  blankinv=off  blankoffset=0  blankwidth=0  evsrcsel=Filtered version of DCAEVT1 (DCAEVT1FILT)  encape=off
  wires:
  Data Type Conversion5/1 -> ePWM5/1
  Constant13/1 -> Saturation Dynamic3/3
  Constant6/1 -> Saturation Dynamic1/1
  Constant12/1 -> Saturation Dynamic3/1
  Constant7/1 -> Saturation Dynamic1/3
  Saturation Dynamic1/1 -> Data Type Conversion5/1
  Constant16/1 -> Saturation Dynamic2/1
  Data Type Conversion18/1 -> ePWM6/1
  Data Type Conversion19/1 -> ePWM7/1
  Saturation Dynamic3/1 -> Data Type Conversion19/1
  Constant17/1 -> Saturation Dynamic2/3
  Saturation Dynamic2/1 -> Data Type Conversion18/1
  PWM1/1 -> Saturation Dynamic1/2
  PWM3/1 -> Saturation Dynamic3/2
  PWM2/1 -> Saturation Dynamic2/2
  From/1 -> ePWM5/2
  From1/1 -> ePWM6/2
  From2/1 -> ePWM7/2
  Trip/1 -> Gain/1
  Gain/1 -> Goto/1

== system Final_Tune_of_Bandwidth_PI_Result/Subsystem1/System Outputs ==

== system Final_Tune_of_Bandwidth_PI_Result/Subsystem3/LPF ==
  u_k : Inport
  Add : Sum  Inputs=+-
  Add1 : Sum
  Delay : Delay  DelayLength=1
  Gain : Gain  Gain=single(100/1100)
  y_k : Outport
  wires:
  Delay/1 -> Add/2, Add1/2
  Add/1 -> Gain/1
  Gain/1 -> Add1/1
  Add1/1 -> y_k/1, Delay/1
  u_k/1 -> Add/1

== system Final_Tune_of_Bandwidth_PI_Result/Subsystem3/LPF1 ==
  u_k : Inport
  Add : Sum  Inputs=+-
  Add1 : Sum
  Delay : Delay  DelayLength=1
  Gain : Gain  Gain=single(100/1100)
  y_k : Outport
  wires:
  Delay/1 -> Add/2, Add1/2
  Add/1 -> Gain/1
  Gain/1 -> Add1/1
  Add1/1 -> y_k/1, Delay/1
  u_k/1 -> Add/1

== system Final_Tune_of_Bandwidth_PI_Result/Subsystem3/LPF2 ==
  u_k : Inport
  Add : Sum  Inputs=+-
  Add1 : Sum
  Delay : Delay  DelayLength=1
  Gain : Gain  Gain=single(100/1100)
  y_k : Outport
  wires:
  Delay/1 -> Add/2, Add1/2
  Add/1 -> Gain/1
  Gain/1 -> Add1/1
  Add1/1 -> y_k/1, Delay/1
  u_k/1 -> Add/1

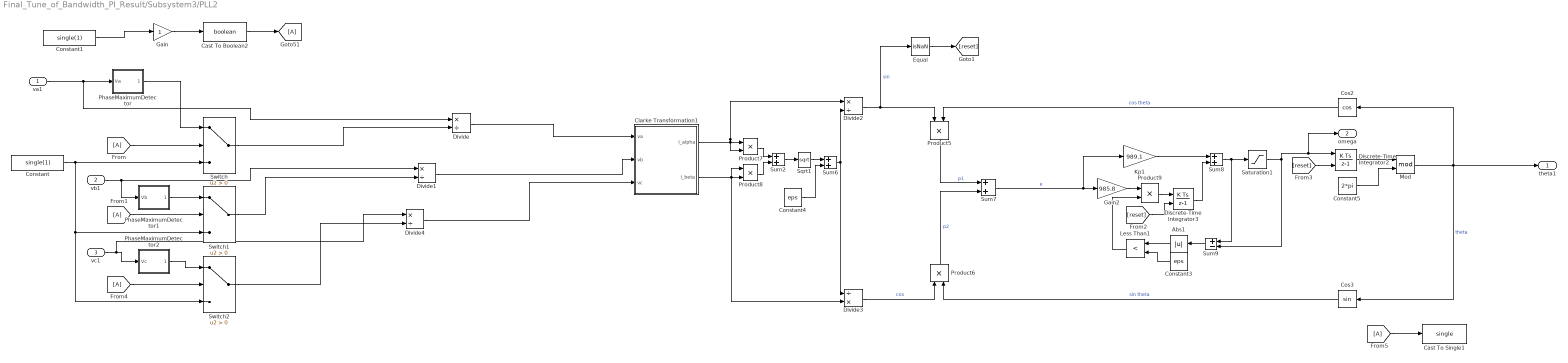
== system Final_Tune_of_Bandwidth_PI_Result/Subsystem3/PLL2 ==
  va1 : Inport
  vb1 : Inport  Port=2
  vc1 : Inport  Port=3
  Abs1 : Abs  SaturateOnIntegerOverflow=off
  Cast To Boolean2 : DataTypeConversion  OutDataTypeStr=boolean  SaturateOnIntegerOverflow=off  RndMeth=Floor
  Cast To Single1 : DataTypeConversion  OutDataTypeStr=single  SaturateOnIntegerOverflow=off  RndMeth=Floor
  Clarke Transformation1 : Subsystem
  Constant : Constant  Value=single(1)
  Constant1 : Constant  Value=single(1)
  Constant3 : Constant  Value=eps  OutDataTypeStr=single  SampleTime=-1
  Constant4 : Constant  Value=eps  OutDataTypeStr=single
  Constant5 : Constant  Value=2*pi  OutDataTypeStr=single  SampleTime=-1
  Cos2 : Trigonometry  Operator=cos
  Cos3 : Trigonometry
  Discrete-Time Integrator2 : DiscreteIntegrator  ExternalReset=either  SampleTime=-1  ICPrevOutput=DiscIntNeverNeededParam  ICPrevScaledInput=DiscIntNeverNeededParam
  Discrete-Time Integrator3 : DiscreteIntegrator  ExternalReset=either  SampleTime=-1  ICPrevOutput=DiscIntNeverNeededParam  ICPrevScaledInput=DiscIntNeverNeededParam
  Divide : Product  Inputs=*/  RndMeth=Zero  SaturateOnIntegerOverflow=on
  Divide1 : Product  Inputs=*/  RndMeth=Zero  SaturateOnIntegerOverflow=on
  Divide2 : Product  Inputs=*/
  Divide3 : Product  Inputs=/*
  Divide4 : Product  Inputs=*/  RndMeth=Zero  SaturateOnIntegerOverflow=on
  Equal : RelationalOperator  Operator=isNaN  OutDataTypeStr=boolean  RndMeth=Simplest  InputSameDT=off
  From{,1,4..5} (4 alike) : From
  Gain : Gain
  Gain2 : Gain  Gain=985.8  SaturateOnIntegerOverflow=on  OutDataTypeStr=Inherit: Same as input  ParamDataTypeStr=Inherit: Same as input
  Goto51 : Goto
  Kp1 : Gain  Gain=989.1  SaturateOnIntegerOverflow=on  OutDataTypeStr=Inherit: Same as input  ParamDataTypeStr=Inherit: Same as input
  Less Than1 : RelationalOperator  Operator=<  OutDataTypeStr=boolean  RndMeth=Simplest  InputSameDT=off
  Mod : Math  Operator=mod
  PhaseMaximumDetector : Subsystem
  PhaseMaximumDetector1 : Subsystem
  PhaseMaximumDetector2 : Subsystem
  Product{5..9} (5 alike) : Product
  Saturation1 : Saturate  UpperLimit=inf  LowerLimit=-inf
  Sqrt1 : Sqrt  OutDataTypeStr=single  IntermediateResultsDataTypeStr=single
  Sum2 : Sum
  Sum6 : Sum  OutDataTypeStr=single
  Sum7 : Sum
  Sum8 : Sum
  Sum9 : Sum  Inputs=+-
  Switch : Switch  Criteria=u2 > Threshold  SaturateOnIntegerOverflow=off  InputSameDT=off
  Switch1 : Switch  Criteria=u2 > Threshold  SaturateOnIntegerOverflow=off  InputSameDT=off
  Switch2 : Switch  Criteria=u2 > Threshold  SaturateOnIntegerOverflow=off  InputSameDT=off
  theta1 : Outport
  omega : Outport  Port=2
  wires:
  Clarke Transformation1/1(I_alpha) -> Divide2/1, Product7/1, Product7/2
  Saturation1/1 -> Sum9/2, omega/1, Discrete-Time Integrator2/1
  Product9/1 -> Discrete-Time Integrator3/1
  Sum9/1 -> Abs1/1
  Abs1/1 -> Less Than1/1
  Cos3/1 -> Product6/2  "sin theta"
  Product7/1 -> Sum2/1
  [reset] -> Discrete-Time Integrator2/2
  Discrete-Time Integrator3/1 -> Sum8/2
  Product8/1 -> Sum2/2
  Divide2/1 -> Product5/1, Equal/1  "sin"
  Product6/1 -> Sum7/2  "p2"
  Sum8/1 -> Sum9/1, Saturation1/1
  Mod/1 -> Cos2/1, theta1/1, Cos3/1  "theta"
  Sum6/1 -> Divide3/1, Divide2/2
  Sum2/1 -> Sqrt1/1
  Divide3/1 -> Product6/1  "cos"
  Clarke Transformation1/2(I_beta) -> Product8/2, Product8/1, Divide3/2
  Cos2/1 -> Product5/2  "cos theta"
  Constant5/1 -> Mod/2
  Product5/1 -> Sum7/1  "p1"
  Sum7/1 -> Kp1/1, Gain2/1  "e"
  Equal/1 -> [reset]
  Kp1/1 -> Sum8/1
  Constant3/1 -> Less Than1/2
  Less Than1/1 -> Product9/2
  [reset] -> Discrete-Time Integrator3/2
  Sqrt1/1 -> Sum6/1
  Gain2/1 -> Product9/1
  Discrete-Time Integrator2/1 -> Mod/1
  Constant4/1 -> Sum6/2
  Divide4/1 -> Clarke Transformation1/3(vc)
  Divide1/1 -> Clarke Transformation1/2(vb)
  Cast To Boolean2/1 -> Goto51/1
  From/1 -> Switch/2
  From1/1 -> Switch1/2
  From4/1 -> Switch2/2
  Constant/1 -> Switch2/3, Switch1/3, Switch/3
  Divide/1 -> Clarke Transformation1/1(va)
  From5/1 -> Cast To Single1/1
  va1/1 -> Divide/1, PhaseMaximumDetector/1(Va)
  PhaseMaximumDetector/1(Vamax) -> Switch/1
  Switch/1 -> Divide/2
  vb1/1 -> Divide1/1, PhaseMaximumDetector1/1(Vb)
  PhaseMaximumDetector1/1(Vbmax) -> Switch1/1
  Switch1/1 -> Divide1/2
  vc1/1 -> Divide4/1, PhaseMaximumDetector2/1(Vc)
  PhaseMaximumDetector2/1(Vcmax) -> Switch2/1
  Switch2/1 -> Divide4/2
  Gain/1 -> Cast To Boolean2/1
  Constant1/1 -> Gain/1

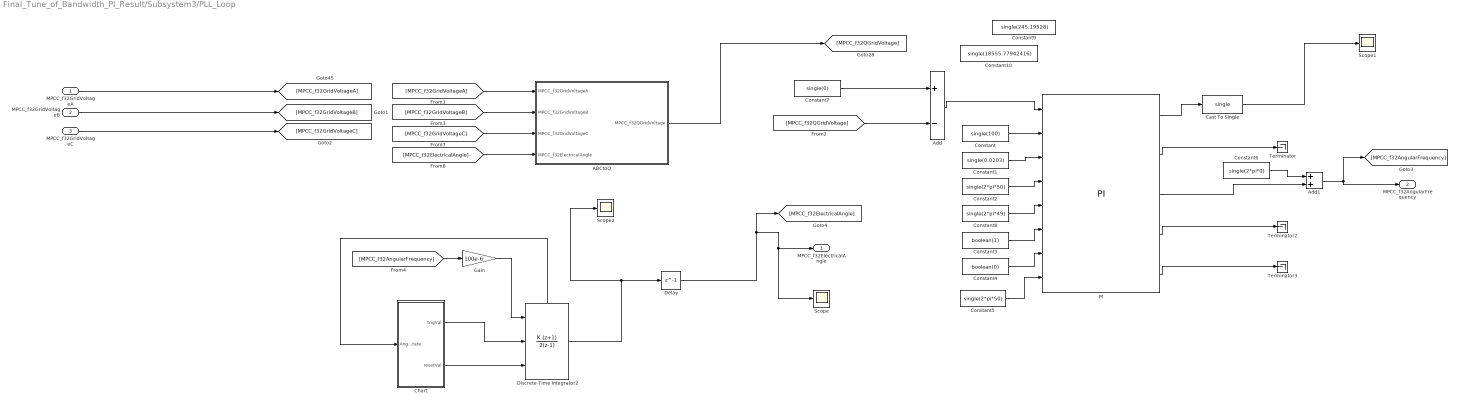
== system Final_Tune_of_Bandwidth_PI_Result/Subsystem3/PLL_Loop ==
  MPCC_f32GridVoltageA : Inport
  MPCC_f32GridVoltageB : Inport  Port=2
  MPCC_f32GridVoltageC : Inport  Port=3
  ABCtoQ : Subsystem
  Add : Sum  Inputs=+-  OutDataTypeStr=Inherit: Inherit via back propagation
  Add1 : Sum
  Cast To Single : DataTypeConversion  OutDataTypeStr=single  SaturateOnIntegerOverflow=off  RndMeth=Floor
  Chart : Stateflow chart  TreatAsAtomicUnit=on
  Constant : Constant  Value=single(100)
  Constant1 : Constant  Value=single(0.0203)
  Constant10 : Constant  Value=single(18555.77942416)
  Constant2 : Constant  Value=single(2*pi*50)
  Constant3 : Constant  Value=boolean(1)
  Constant4 : Constant  Value=boolean(0)
  Constant5 : Constant  Value=single(2*pi*50)
  Constant6 : Constant  Value=single(2*pi*0)
  Constant7 : Constant  Value=single(0)
  Constant8 : Constant  Value=single(2*pi*49)
  Constant9 : Constant  Value=single(245.19528)
  Delay : Delay  DelayLength=1
  Discrete-Time Integrator2 : DiscreteIntegrator  IntegratorMethod=Accumulation: Trapezoidal  ExternalReset=sampled level  InitialConditionSource=external  SampleTime=-1  ShowStatePort=on  ICPrevOutput=DiscIntNeverNeededParam  ICPrevScaledInput=DiscIntNeverNeededParam
  Gain : Gain  Gain=100e-6
  PI : PID_Lib/PI  SystemSampleTime=-1  VariantActivationTime=update diagram  Latency=0  AutoFrameSizeCalculation=off
  Scope : Scope
  Scope1 : Scope
  Scope2 : Scope
  Terminator : Terminator
  Terminator2 : Terminator
  Terminator3 : Terminator
  MPCC_f32ElectricalAngle : Outport
  MPCC_f32AngularFrequency : Outport  Port=2
  wires:
  Constant7/1 -> Add/1
  PI/2 -> Terminator/1
  PI/4 -> Terminator2/1
  PI/5 -> Terminator3/1
  MPCC_f32GridVoltageB/1 -> [MPCC_f32GridVoltageB]
  MPCC_f32GridVoltageC/1 -> [MPCC_f32GridVoltageC]
  [MPCC_f32GridVoltageC] -> ABCtoQ/3(MPCC_f32GridVoltageC)
  [MPCC_f32ElectricalAngle] -> ABCtoQ/4(MPCC_f32ElectricalAngle)
  [MPCC_f32GridVoltageA] -> ABCtoQ/1(MPCC_f32GridVoltageA)
  [MPCC_f32QGridVoltage] -> Add/2
  PI/1 -> Cast To Single/1
  Cast To Single/1 -> Scope1/1
  Discrete-Time Integrator2/1 -> Scope2/1, Delay/1
  [MPCC_f32AngularFrequency] -> Gain/1
  Discrete-Time Integrator2/State -> Chart/1(Angle_State)
  Chart/1(trigVal) -> Discrete-Time Integrator2/2
  Chart/2(resetVal) -> Discrete-Time Integrator2/3
  Gain/1 -> Discrete-Time Integrator2/1
  [MPCC_f32GridVoltageB] -> ABCtoQ/2(MPCC_f32GridVoltageB)
  Add/1 -> PI/1
  Constant2/1 -> PI/4
  Constant8/1 -> PI/5
  Constant3/1 -> PI/6
  Constant4/1 -> PI/7
  MPCC_f32GridVoltageA/1 -> [MPCC_f32GridVoltageA]
  Constant5/1 -> PI/8
  Delay/1 -> [MPCC_f32ElectricalAngle], Scope/1, MPCC_f32ElectricalAngle/1
  ABCtoQ/1(MPCC_f32QGridVoltage) -> [MPCC_f32QGridVoltage]
  Constant6/1 -> Add1/1
  Add1/1 -> [MPCC_f32AngularFrequency], MPCC_f32AngularFrequency/1
  Constant/1 -> PI/2
  Constant1/1 -> PI/3
  PI/3 -> Add1/2

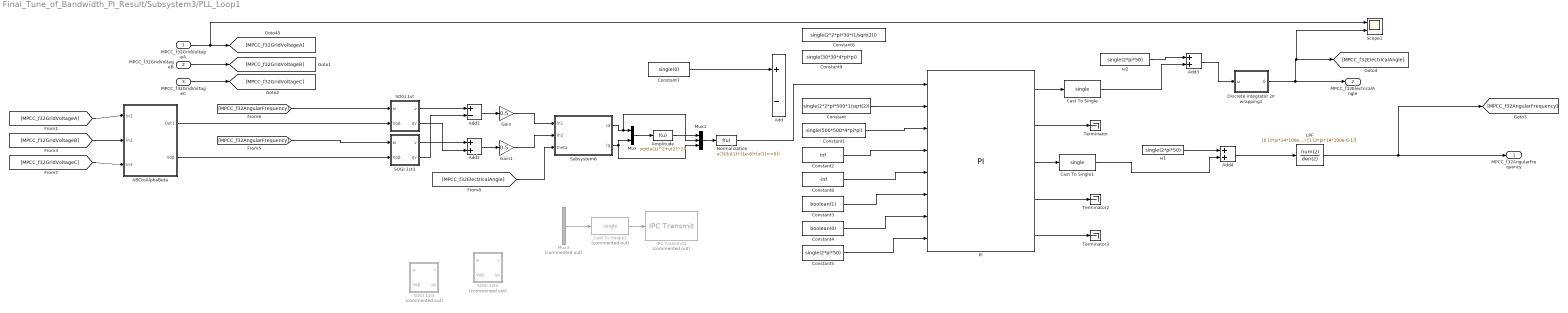
== system Final_Tune_of_Bandwidth_PI_Result/Subsystem3/PLL_Loop1 ==
  MPCC_f32GridVoltageA : Inport
  MPCC_f32GridVoltageB : Inport  Port=2
  MPCC_f32GridVoltageC : Inport  Port=3
  ABCtoAlphaBeta : Subsystem
  Add : Sum  Inputs=+-  OutDataTypeStr=Inherit: Inherit via back propagation
  Add1 : Sum  Inputs=+-
  Add2 : Sum
  Add3 : Sum
  Add4 : Sum
  Amplitude : Fcn  Expr=sqrt(u(1)^2+u(2)^2)
  Cast To Single : DataTypeConversion  OutDataTypeStr=single  SaturateOnIntegerOverflow=off  RndMeth=Floor
  Cast To Single1 : DataTypeConversion  OutDataTypeStr=single  SaturateOnIntegerOverflow=off  RndMeth=Floor
  Cast To Single2 : DataTypeConversion  Commented=on  OutDataTypeStr=single  SaturateOnIntegerOverflow=off  RndMeth=Floor
  Constant : Constant  Value=single(2*2*pi*500*1/sqrt(2))  VectorParams1D=off
  Constant1 : Constant  Value=single(500*500*4*pi*pi)
  Constant2 : Constant  Value=inf
  Constant3 : Constant  Value=boolean(1)
  Constant4 : Constant  Value=boolean(0)
  Constant5 : Constant  Value=single(2*pi*50)
  Constant6 : Constant  Value=single(2*2*pi*30*(1/sqrt(2)))
  Constant7 : Constant  Value=single(0)
  Constant8 : Constant  Value=-inf
  Constant9 : Constant  Value=single(30*30*4*pi*pi)
  Discrete integrator 2π wrapping1 : Subsystem
  Gain : Gain  Gain=0.5
  Gain1 : Gain  Gain=0.5
  IPC Transmit2 : c2837xDlib/IPC Transmit  Commented=on  blkParamProc=F2837x  SelectDestination=C28x (CPU1/CPU2)  SelectChannel=0  EnableBlocking=off
  LPF : DiscreteFilter  Numerator=[0 (2*pi*14*100e-6)]  Denominator=[1 (2*pi*14*100e-6-1)]  InitialStates=50/14/100e-6
  Mux : Mux  Inputs=2
  Mux1 : Mux  Inputs=3
  Mux4 : Mux  Commented=on  Inputs=3
  Normalization : Fcn  Expr=u(3)/(u(1)+(1e-6)*(u(1)==0))
  PI : PID_Lib/PI  SystemSampleTime=-1  VariantActivationTime=update diagram  Latency=0  AutoFrameSizeCalculation=off
  SOGI 1st : Subsystem
  SOGI 1st2 : Subsystem  Commented=on
  SOGI 1st3 : Subsystem
  SOGI 1st4 : Subsystem  Commented=on
  Scope1 : Scope  NumInputPorts=2
  Subsystem6 : Subsystem
  Terminator : Terminator
  Terminator2 : Terminator
  Terminator3 : Terminator
  ω1 : Constant  Value=single(2*pi*50)  OutDataTypeStr=single
  ω2 : Constant  Value=single(2*pi*50)  OutDataTypeStr=single
  MPCC_f32AngularFrequency : Outport
  MPCC_f32ElectricalAngle : Outport  Port=2
  wires:
  Constant7/1 -> Add/1
  Constant2/1 -> PI/4
  Constant3/1 -> PI/6
  Constant4/1 -> PI/7
  PI/2 -> Terminator/1
  PI/4 -> Terminator2/1
  PI/5 -> Terminator3/1
  MPCC_f32GridVoltageB/1 -> [MPCC_f32GridVoltageB]
  MPCC_f32GridVoltageC/1 -> [MPCC_f32GridVoltageC]
  Constant8/1 -> PI/5
  PI/1 -> Cast To Single/1
  [MPCC_f32GridVoltageA] -> ABCtoAlphaBeta/1(In1)
  [MPCC_f32GridVoltageB] -> ABCtoAlphaBeta/2(In2)
  [MPCC_f32GridVoltageC] -> ABCtoAlphaBeta/3(In3)
  Add1/1 -> Gain/1
  Add2/1 -> Gain1/1
  Gain/1 -> Subsystem6/1(In1)
  Gain1/1 -> Subsystem6/2(In2)
  Constant5/1 -> PI/8
  Subsystem6/1(Id) -> Mux1/2, Mux/1
  Subsystem6/2(Iq) -> Mux1/3, Mux/2
  Mux/1 -> Amplitude/1
  Mux1/1 -> Normalization/1
  Amplitude/1 -> Mux1/1
  Cast To Single/1 -> Add3/2
  ω2/1 -> Add3/1
  Add3/1 -> Discrete integrator 2π wrapping1/1(ω)
  Discrete integrator 2π wrapping1/1(θ) -> Scope1/2, [MPCC_f32ElectricalAngle], MPCC_f32ElectricalAngle/1
  PI/3 -> Cast To Single1/1
  ω1/1 -> Add4/1
  Cast To Single1/1 -> Add4/2
  [MPCC_f32ElectricalAngle] -> Subsystem6/3(theta)
  Add4/1 -> LPF/1
  [MPCC_f32AngularFrequency] -> SOGI 1st/1(w)
  [MPCC_f32AngularFrequency] -> SOGI 1st3/1(w)
  MPCC_f32GridVoltageA/1 -> Scope1/1, [MPCC_f32GridVoltageA]
  Normalization/1 -> PI/1
  Constant/1 -> PI/2
  Constant1/1 -> PI/3
  LPF/1 -> [MPCC_f32AngularFrequency], MPCC_f32AngularFrequency/1
  ABCtoAlphaBeta/1(Out1) -> SOGI 1st/2(Vαβ)
  ABCtoAlphaBeta/2(Vαβ) -> SOGI 1st3/2(Vαβ)
  SOGI 1st/1(v) -> Add1/1
  SOGI 1st/2(qv) -> Add2/2
  SOGI 1st3/2(qv) -> Add1/2
  SOGI 1st3/1(v) -> Add2/1
  Cast To Single2/1 -> IPC Transmit2/1
  Mux4/1 -> Cast To Single2/1

== system Final_Tune_of_Bandwidth_PI_Result/Subsystem3/RateLimiter ==
  Up : Inport
  Ts : Inport  Port=2
  Lo : Inport  Port=3
  U : Inport  Port=4
  Xo : Inport  Port=5
  Rs : Inport  Port=6
  Add1 : Sum  Inputs=+-
  Add2 : Sum
  Data Type Duplicate : DataTypeDuplicate  NumInputPorts=7
  Delay : Delay  DelayLength=1  InitialConditionSource=Input port  ExternalReset=Rising
      settings: InputPortMap=u0,r5,p4
  Product : Product
  Product1 : Product
  Saturation Dynamic : simulink/Discontinuities/Saturation Dynamic  OutMin=[]  OutMax=[]  OutDataTypeStr=Inherit: Same as second input  OutDataType=fixdt(1, 16)  OutScaling=2^-10  DoSatur=off
  Y : Outport
  wires:
  Xo/1 -> Delay/3
  Product1/1 -> Data Type Duplicate/3, Saturation Dynamic/3
  Add1/1 -> Data Type Duplicate/4, Saturation Dynamic/2
  Add2/1 -> Data Type Duplicate/1, Y/1, Delay/1
  Delay/1 -> Data Type Duplicate/2, Add1/2, Add2/2
  U/1 -> Data Type Duplicate/5, Add1/1
  Saturation Dynamic/1 -> Data Type Duplicate/7, Add2/1
  Product/1 -> Data Type Duplicate/6, Saturation Dynamic/1
  Rs/1 -> Delay/2
  Ts/1 -> Product1/1, Product/2
  Lo/1 -> Product1/2
  Up/1 -> Product/1

== system Final_Tune_of_Bandwidth_PI_Result/Subsystem3/RateLimiter1 ==
  Up : Inport
  Ts : Inport  Port=2
  Lo : Inport  Port=3
  U : Inport  Port=4
  Xo : Inport  Port=5
  Rs : Inport  Port=6
  Add1 : Sum  Inputs=+-
  Add2 : Sum
  Data Type Duplicate : DataTypeDuplicate  NumInputPorts=7
  Delay : Delay  DelayLength=1  InitialConditionSource=Input port  ExternalReset=Rising
      settings: InputPortMap=u0,r5,p4
  Product : Product
  Product1 : Product
  Saturation Dynamic : simulink/Discontinuities/Saturation Dynamic  OutMin=[]  OutMax=[]  OutDataTypeStr=Inherit: Same as second input  OutDataType=fixdt(1, 16)  OutScaling=2^-10  DoSatur=off
  Y : Outport
  wires:
  Xo/1 -> Delay/3
  Product1/1 -> Data Type Duplicate/3, Saturation Dynamic/3
  Add1/1 -> Data Type Duplicate/4, Saturation Dynamic/2
  Add2/1 -> Data Type Duplicate/1, Y/1, Delay/1
  Delay/1 -> Data Type Duplicate/2, Add1/2, Add2/2
  U/1 -> Data Type Duplicate/5, Add1/1
  Saturation Dynamic/1 -> Data Type Duplicate/7, Add2/1
  Product/1 -> Data Type Duplicate/6, Saturation Dynamic/1
  Rs/1 -> Delay/2
  Ts/1 -> Product1/1, Product/2
  Lo/1 -> Product1/2
  Up/1 -> Product/1

== system Final_Tune_of_Bandwidth_PI_Result/Subsystem3/RateLimiter2 ==
  Up : Inport
  Ts : Inport  Port=2
  Lo : Inport  Port=3
  U : Inport  Port=4
  Xo : Inport  Port=5
  Rs : Inport  Port=6
  Add1 : Sum  Inputs=+-
  Add2 : Sum
  Data Type Duplicate : DataTypeDuplicate  NumInputPorts=7
  Delay : Delay  DelayLength=1  InitialConditionSource=Input port  ExternalReset=Rising
      settings: InputPortMap=u0,r5,p4
  Product : Product
  Product1 : Product
  Saturation Dynamic : simulink/Discontinuities/Saturation Dynamic  OutMin=[]  OutMax=[]  OutDataTypeStr=Inherit: Same as second input  OutDataType=fixdt(1, 16)  OutScaling=2^-10  DoSatur=off
  Y : Outport
  wires:
  Xo/1 -> Delay/3
  Product1/1 -> Data Type Duplicate/3, Saturation Dynamic/3
  Add1/1 -> Data Type Duplicate/4, Saturation Dynamic/2
  Add2/1 -> Data Type Duplicate/1, Y/1, Delay/1
  Delay/1 -> Data Type Duplicate/2, Add1/2, Add2/2
  U/1 -> Data Type Duplicate/5, Add1/1
  Saturation Dynamic/1 -> Data Type Duplicate/7, Add2/1
  Product/1 -> Data Type Duplicate/6, Saturation Dynamic/1
  Rs/1 -> Delay/2
  Ts/1 -> Product1/1, Product/2
  Lo/1 -> Product1/2
  Up/1 -> Product/1
